simulink model "online_block"  (R2024b)
settings: Solver=VariableStepAuto  StartTime=0.0  StopTime=1000.0  RelTol=1e-3
settings Model: Creator=klyx  LastModifiedBy=klyx

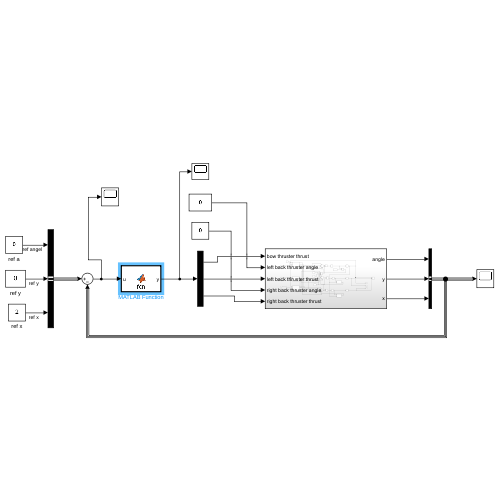
[thumbnail: Simulink's stored preview of the top-level diagram]
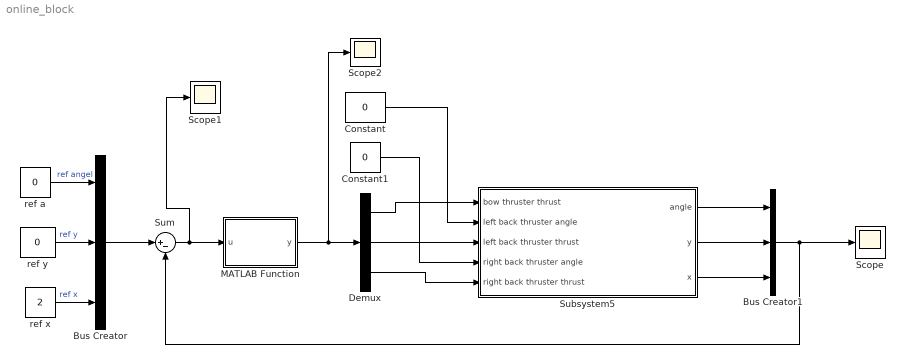
== system online_block ==
  Bus Creator : BusCreator  Inputs=3
  Bus Creator1 : BusCreator  Inputs=3
  Constant : Constant  Value=0
  Constant1 : Constant  Value=0
  Demux : Demux  Outputs=3
  MATLAB Function : MATLAB Function  TreatAsAtomicUnit=on
  Scope : Scope
  Scope1 : Scope
  Scope2 : Scope
  Subsystem5 : Subsystem
  Sum : Sum  Inputs=|+-
  ref a : Constant  Value=0
  ref x : Constant  Value=2
  ref y : Constant  Value=0
  wires:
  Constant/1 -> Subsystem5/2(left back thruster angle)
  Constant1/1 -> Subsystem5/4(right back thruster angle)
  Subsystem5/1(angle) -> Bus Creator1/1
  Subsystem5/2(y) -> Bus Creator1/2
  Subsystem5/3(x) -> Bus Creator1/3
  ref a/1 -> Bus Creator/1  "ref angel"
  Bus Creator/1 -> Sum/1
  Bus Creator1/1 -> Scope/1, Sum/2
  MATLAB Function/1(y) -> Scope2/1, Demux/1
  Demux/1 -> Subsystem5/1("bow thruster thrust ")
  Demux/2 -> Subsystem5/3(left back thruster thrust)
  Demux/3 -> Subsystem5/5(right back thruster thrust)
  Sum/1 -> Scope1/1, MATLAB Function/1(u)
  ref y/1 -> Bus Creator/2  "ref y"
  ref x/1 -> Bus Creator/3  "ref x"

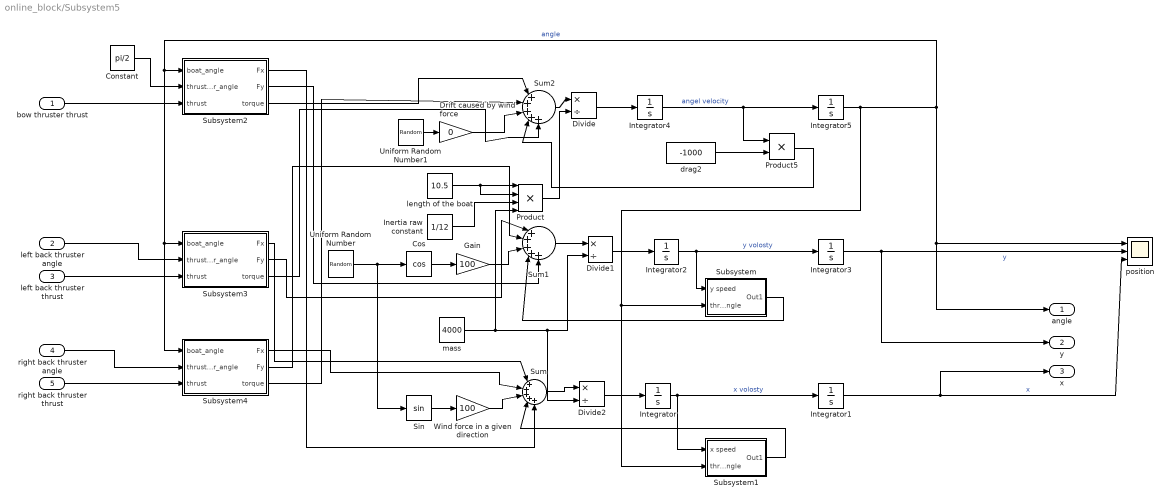
== system online_block/Subsystem5 ==
  "bow thruster thrust " : Inport
  left back thruster angle : Inport  Port=2
  left back thruster thrust : Inport  Port=3
  right back thruster angle : Inport  Port=4
  right back thruster thrust : Inport  Port=5
  Constant : Constant  Value=pi/2
  Cos : Trigonometry  Operator=cos
  Divide : Product  Inputs=*/
  Divide1 : Product  Inputs=*/
  Divide2 : Product  Inputs=*/
  Drift caused by wind force : Gain  Gain=0
  Gain : Gain  Gain=100
  Inertia raw constant : Constant  Value=1/12
  Integrator{,1..5} (6 alike) : Integrator
  Product : Product  Inputs=4
  Product5 : Product
  Sin : Trigonometry
  Subsystem : Subsystem
  Subsystem1 : Subsystem
  Subsystem2 : Subsystem
  Subsystem3 : Subsystem
  Subsystem4 : Subsystem
  Sum : Sum  Inputs=|+++++
  Sum1 : Sum  Inputs=|+++++
  Sum2 : Sum  Inputs=|+++++
  Uniform Random Number : UniformRandomNumber  Minimum=0  Maximum=6.28  Seed=0.1  SampleTime=0.1
  Uniform Random Number1 : UniformRandomNumber  Seed=2  SampleTime=0.1
  Wind force in a given direction : Gain  Gain=100
  drag2 : Constant  Value=-1000
  length of the boat : Constant  Value=10.5
  mass : Constant  Value=4000
  position : Scope  NumInputPorts=3
  angle : Outport
  y : Outport  Port=2
  x : Outport  Port=3
  wires:
  Sum2/1 -> Divide/1
  Subsystem/1(Out1) -> Sum1/4
  Product/1 -> Divide/2
  Sum/1 -> Divide2/1
  Subsystem3/2(Fy) -> Sum1/1
  Subsystem4/3(torque) -> Sum2/2
  Subsystem2/3(torque) -> Sum2/1
  Subsystem1/1(Out1) -> Sum/4
  Subsystem2/2(Fy) -> Sum1/5
  Subsystem4/2(Fy) -> Sum1/2
  Divide1/1 -> Integrator2/1
  drag2/1 -> Product5/2
  Sum1/1 -> Divide1/1
  Product5/1 -> Sum2/4
  Sin/1 -> Wind force in a given direction/1
  Gain/1 -> Sum1/3
  Drift caused by wind force/1 -> Sum2/3
  Integrator5/1 -> Subsystem1/2(thruster angle), Subsystem/2(thruster angle), angle/1, position/1, Subsystem2/1(boat_angle), Subsystem4/1(boat_angle), Subsystem3/1(boat_angle)  "angle"
  "bow thruster thrust "/1 -> Subsystem2/3(thrust)
  Subsystem3/1(Fx) -> Sum/1
  right back thruster thrust/1 -> Subsystem4/3(thrust)
  Divide2/1 -> Integrator/1
  Integrator3/1 -> y/1, position/2  "y"
  Divide/1 -> Integrator4/1
  Integrator1/1 -> x/1, position/3  "x"
  Subsystem2/1(Fx) -> Sum/5
  Integrator/1 -> Subsystem1/1(x speed), Integrator1/1  "x volosty"
  right back thruster angle/1 -> Subsystem4/2(thruster_angle)
  length of the boat/1 -> Product/2, Product/1
  Constant/1 -> Subsystem2/2(thruster_angle)
  left back thruster thrust/1 -> Subsystem3/3(thrust)
  Subsystem3/3(torque) -> Sum2/5
  Subsystem4/1(Fx) -> Sum/2
  Integrator2/1 -> Subsystem/1(y speed), Integrator3/1  "y volosty"
  left back thruster angle/1 -> Subsystem3/2(thruster_angle)
  Cos/1 -> Gain/1
  Integrator4/1 -> Product5/1, Integrator5/1  "angel velocity"
  Uniform Random Number1/1 -> Drift caused by wind force/1
  Uniform Random Number/1 -> Sin/1, Cos/1
  Wind force in a given direction/1 -> Sum/3
  mass/1 -> Product/4, Divide2/2, Divide1/2
  Inertia raw constant/1 -> Product/3

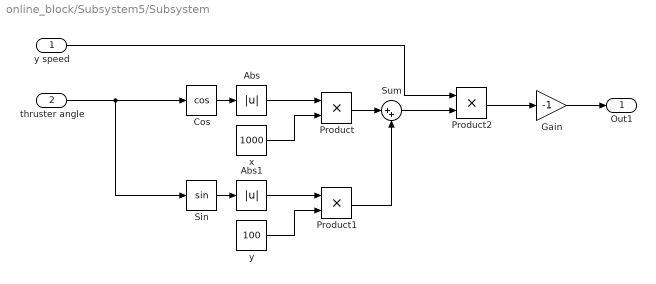
== system online_block/Subsystem5/Subsystem ==
  y speed : Inport
  thruster angle : Inport  Port=2
  Abs : Abs  SaturateOnIntegerOverflow=off
  Abs1 : Abs  SaturateOnIntegerOverflow=off
  Cos : Trigonometry  Operator=cos
  Gain : Gain  Gain=-1
  Product : Product
  Product1 : Product
  Product2 : Product
  Sin : Trigonometry
  Sum : Sum  Inputs=|++
  x : Constant  Value=1000
  y : Constant  Value=100
  Out1 : Outport
  wires:
  Product1/1 -> Sum/2
  Abs1/1 -> Product1/1
  Abs/1 -> Product/1
  Cos/1 -> Abs/1
  Product2/1 -> Gain/1
  Gain/1 -> Out1/1
  thruster angle/1 -> Sin/1, Cos/1
  Product/1 -> Sum/1
  x/1 -> Product/2
  y/1 -> Product1/2
  Sum/1 -> Product2/2
  Sin/1 -> Abs1/1
  y speed/1 -> Product2/1

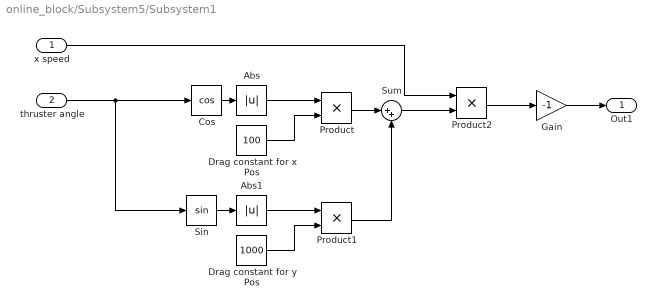
== system online_block/Subsystem5/Subsystem1 ==
  x speed : Inport
  thruster angle : Inport  Port=2
  Abs : Abs  SaturateOnIntegerOverflow=off
  Abs1 : Abs  SaturateOnIntegerOverflow=off
  Cos : Trigonometry  Operator=cos
  Drag constant for x Pos : Constant  Value=100
  Drag constant for y Pos : Constant  Value=1000
  Gain : Gain  Gain=-1
  Product : Product
  Product1 : Product
  Product2 : Product
  Sin : Trigonometry
  Sum : Sum  Inputs=|++
  Out1 : Outport
  wires:
  Product1/1 -> Sum/2
  Abs1/1 -> Product1/1
  Abs/1 -> Product/1
  Cos/1 -> Abs/1
  Product2/1 -> Gain/1
  Gain/1 -> Out1/1
  thruster angle/1 -> Sin/1, Cos/1
  Product/1 -> Sum/1
  Drag constant for x Pos/1 -> Product/2
  Drag constant for y Pos/1 -> Product1/2
  Sum/1 -> Product2/2
  Sin/1 -> Abs1/1
  x speed/1 -> Product2/1

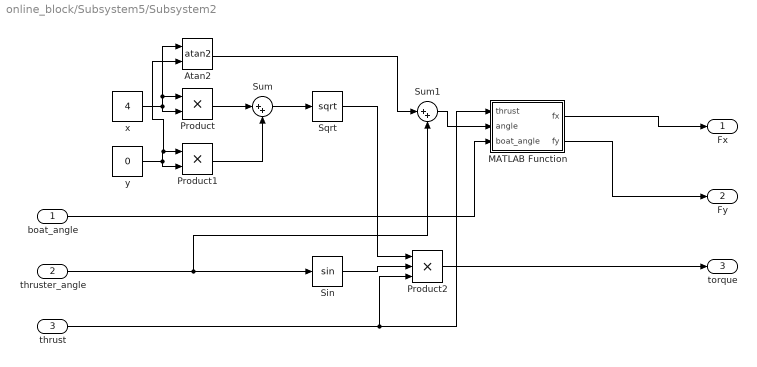
== system online_block/Subsystem5/Subsystem2 ==
  boat_angle : Inport
  thruster_angle : Inport  Port=2
  thrust : Inport  Port=3
  Atan2 : Trigonometry  Operator=atan2
  MATLAB Function : MATLAB Function  TreatAsAtomicUnit=on
  Product : Product
  Product1 : Product
  Product2 : Product  Inputs=3
  Sin : Trigonometry
  Sqrt : Sqrt
  Sum : Sum  Inputs=|++
  Sum1 : Sum  Inputs=|++
  x : Constant  Value=4
  y : Constant  Value=0
  Fx : Outport
  Fy : Outport  Port=2
  torque : Outport  Port=3
  wires:
  Sin/1 -> Product2/2
  Product1/1 -> Sum/2
  y/1 -> Product1/2, Atan2/2, Product1/1
  Product/1 -> Sum/1
  thruster_angle/1 -> Sum1/2, Sin/1
  thrust/1 -> MATLAB Function/1(thrust), Product2/3
  boat_angle/1 -> MATLAB Function/3(boat_angle)
  MATLAB Function/1(fx) -> Fx/1
  MATLAB Function/2(fy) -> Fy/1
  Sum/1 -> Sqrt/1
  Product2/1 -> torque/1
  Sqrt/1 -> Product2/1
  x/1 -> Atan2/1, Product/1, Product/2
  Atan2/1 -> Sum1/1
  Sum1/1 -> MATLAB Function/2(angle)

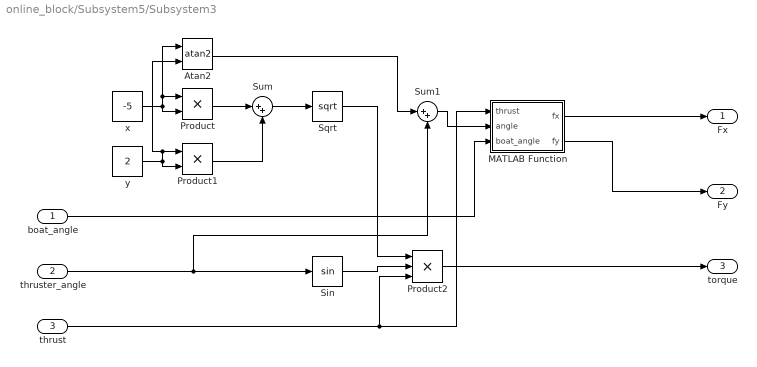
== system online_block/Subsystem5/Subsystem3 ==
  boat_angle : Inport
  thruster_angle : Inport  Port=2
  thrust : Inport  Port=3
  Atan2 : Trigonometry  Operator=atan2
  MATLAB Function : MATLAB Function  TreatAsAtomicUnit=on
  Product : Product
  Product1 : Product
  Product2 : Product  Inputs=3
  Sin : Trigonometry
  Sqrt : Sqrt
  Sum : Sum  Inputs=|++
  Sum1 : Sum  Inputs=|++
  x : Constant  Value=-5
  y : Constant  Value=2
  Fx : Outport
  Fy : Outport  Port=2
  torque : Outport  Port=3
  wires:
  Sin/1 -> Product2/2
  Product1/1 -> Sum/2
  y/1 -> Product1/2, Product1/1, Atan2/2
  Product/1 -> Sum/1
  thruster_angle/1 -> Sum1/2, Sin/1
  thrust/1 -> MATLAB Function/1(thrust), Product2/3
  boat_angle/1 -> MATLAB Function/3(boat_angle)
  MATLAB Function/1(fx) -> Fx/1
  MATLAB Function/2(fy) -> Fy/1
  Sum/1 -> Sqrt/1
  Product2/1 -> torque/1
  Sqrt/1 -> Product2/1
  x/1 -> Atan2/1, Product/1, Product/2
  Atan2/1 -> Sum1/1
  Sum1/1 -> MATLAB Function/2(angle)

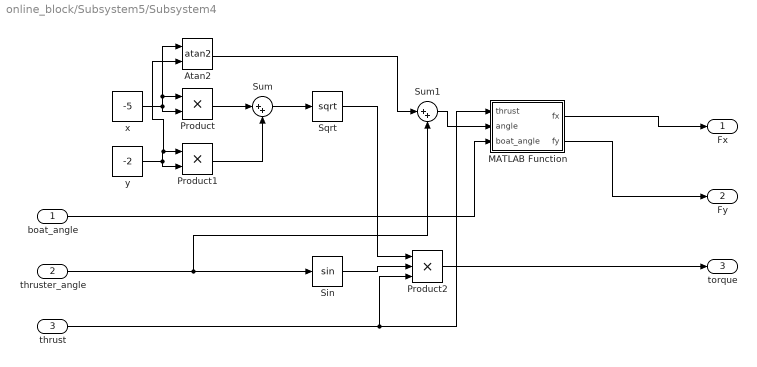
== system online_block/Subsystem5/Subsystem4 ==
  boat_angle : Inport
  thruster_angle : Inport  Port=2
  thrust : Inport  Port=3
  Atan2 : Trigonometry  Operator=atan2
  MATLAB Function : MATLAB Function  TreatAsAtomicUnit=on
  Product : Product
  Product1 : Product
  Product2 : Product  Inputs=3
  Sin : Trigonometry
  Sqrt : Sqrt
  Sum : Sum  Inputs=|++
  Sum1 : Sum  Inputs=|++
  x : Constant  Value=-5
  y : Constant  Value=-2
  Fx : Outport
  Fy : Outport  Port=2
  torque : Outport  Port=3
  wires:
  Sin/1 -> Product2/2
  Product1/1 -> Sum/2
  y/1 -> Product1/2, Atan2/2, Product1/1
  Product/1 -> Sum/1
  thruster_angle/1 -> Sum1/2, Sin/1
  thrust/1 -> MATLAB Function/1(thrust), Product2/3
  boat_angle/1 -> MATLAB Function/3(boat_angle)
  MATLAB Function/1(fx) -> Fx/1
  MATLAB Function/2(fy) -> Fy/1
  Sum/1 -> Sqrt/1
  Product2/1 -> torque/1
  Sqrt/1 -> Product2/1
  x/1 -> Atan2/1, Product/1, Product/2
  Atan2/1 -> Sum1/1
  Sum1/1 -> MATLAB Function/2(angle)

== matlab function online_block/Subsystem5/Subsystem3/MATLAB Function ==
  data: thrust input; fx output; angle input; boat_angle input; fy output
function [fx,fy] = fcn(thrust, angle, boat_angle)

Rx = [cos(boat_angle) -sin(boat_angle); sin(boat_angle) cos(boat_angle)];
f = [sin(angle); cos(angle)];
mf = (Rx*f)*thrust*(-1);
fx = mf(1);
fy = mf(2);

== matlab function online_block/Subsystem5/Subsystem2/MATLAB Function ==
  data: thrust input; fx output; angle input; boat_angle input; fy output
function [fx,fy] = fcn(thrust, angle, boat_angle)

Rx = [cos(boat_angle) -sin(boat_angle); sin(boat_angle) cos(boat_angle)];
f = [sin(angle); cos(angle)];
mf = (Rx*f)*thrust;
fx = mf(1);
fy = mf(2);

== matlab function online_block/Subsystem5/Subsystem4/MATLAB Function ==
  data: thrust input; fx output; angle input; boat_angle input; fy output
function [fx,fy] = fcn(thrust, angle, boat_angle)

Rx = [cos(boat_angle) -sin(boat_angle); sin(boat_angle) cos(boat_angle)];
f = [sin(angle); cos(angle)];
mf = (Rx*f)*thrust*(-1);
fx = mf(1);
fy = mf(2);

== matlab function online_block/MATLAB Function ==
  data: u input; y output
function y = fcn(u)

c = 5000.5;
A = [ 0 0 0; 0 0 1; 0 0 1]*c;

theta_1 = 1;
moter_1_x = -2;
moter_1_y = -5;
len_origen_1 = sqrt(moter_1_y*moter_1_y + moter_1_x*moter_1_x);
vector_angel_1 = atan2(moter_1_y, moter_1_y);

theta_2 = 1;
moter_2_x = 2;
moter_2_y = -5;
len_origen_2 = sqrt(moter_1_y*moter_1_y + moter_1_x*moter_1_x);
vector_angel_2 = atan2(moter_1_y, moter_1_y);

theta_3 = 1;
moter_1_3 = 0;
moter_1_3 = 4;
len_origen_3 = sqrt(moter_1_y*moter_1_y + moter_1_x*moter_1_x);
vector_angel_3 = atan2(moter_1_y, moter_1_y);

%u = [t_1; t_2; t_3];
B = [cos(theta_1+vector_angel_1), cos(theta_2+vector_angel_2) 0;
     sin(theta_1+vector_angel_1) sin(theta_2+vector_angel_2) 1;
     sin(theta_1)*len_origen_1 sin(theta_2)*len_origen_2 sin(theta_3)*len_origen_3]

%y = [0 0 2];
y = A*u;
